simulink model "Quad_Nonlinear_Yaw_PID"  (R2020a)
settings: Solver=ode4  StartTime=0.0  StopTime=10  FixedStep=0.01  RelTol=1e-3
InitFcn:
  | QuadConstants;
undefined symbols (not defined in the file or in its folder): C1, C2, C3, KD_Yaw, KI_Yaw, KP_Yaw, magnitude
libraries: simulink x1
settings Model: Creator=Ali  LastModifiedBy=Ali

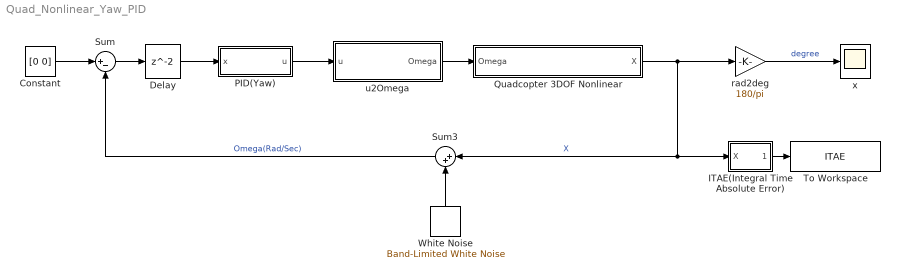
== system Quad_Nonlinear_Yaw_PID ==
  " White Noise" : simulink/Sources/Band-Limited White Noise  Cov=[0.000005]  Ts=.01  seed=[23341]
  Constant : Constant  Value=[0 0]
  Delay : Delay
  ITAE(Integral Time Absolute Error) : Subsystem
  PID(Yaw) : Subsystem
  Quadcopter 3DOF Nonlinear : Subsystem  TreatAsAtomicUnit=on
  Sum : Sum  Inputs=|+-
  Sum3 : Sum  Inputs=|++
  To Workspace : ToWorkspace  VariableName=ITAE  SaveFormat=Timeseries  SampleTime=-1
  rad2deg : Gain  Gain=180/pi
  u2Omega : Subsystem
  x : Scope
  wires:
  Quadcopter 3DOF Nonlinear/1(X) -> Sum3/1, ITAE(Integral Time Absolute Error)/1(X), rad2deg/1  "X"
  ITAE(Integral Time Absolute Error)/1(ITAE) -> To Workspace/1
  " White Noise"/1 -> Sum3/2
  rad2deg/1 -> x/1  "degree"
  Sum3/1 -> Sum/2  "Omega(Rad/Sec)"
  u2Omega/1(Omega) -> Quadcopter 3DOF Nonlinear/1(Omega)
  Constant/1 -> Sum/1
  PID(Yaw)/1(u) -> u2Omega/1(u)
  Sum/1 -> Delay/1
  Delay/1 -> PID(Yaw)/1(x)

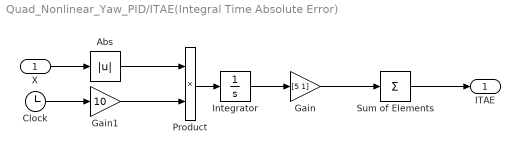
== system Quad_Nonlinear_Yaw_PID/ITAE(Integral Time Absolute Error) ==
  X : Inport
  Abs : Abs
  Clock : Clock
  Gain : Gain  Gain=[5 1]
  Gain1 : Gain  Gain=10
  Integrator : Integrator
  Product : Product
  Sum of Elements : Sum  Inputs=+
  ITAE : Outport
  wires:
  Product/1 -> Integrator/1
  Integrator/1 -> Gain/1
  Clock/1 -> Gain1/1
  Sum of Elements/1 -> ITAE/1
  Abs/1 -> Product/1
  X/1 -> Abs/1
  Gain/1 -> Sum of Elements/1
  Gain1/1 -> Product/2

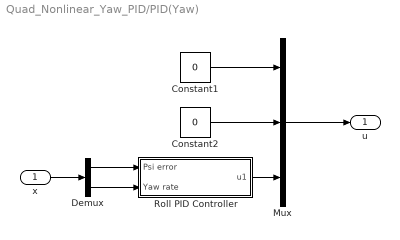
== system Quad_Nonlinear_Yaw_PID/PID(Yaw) ==
  x : Inport
  Constant1 : Constant  Value=0
  Constant2 : Constant  Value=0
  Demux : Demux  Outputs=2
  Mux : Mux  Inputs=3
  Roll PID Controller : Subsystem  VariantControl=Choice
  u : Outport
  wires:
  Mux/1 -> u/1
  x/1 -> Demux/1
  Demux/2 -> Roll PID Controller/2(Yaw rate)
  Demux/1 -> Roll PID Controller/1(Psi error)
  Constant1/1 -> Mux/1
  Roll PID Controller/1(u1) -> Mux/3
  Constant2/1 -> Mux/2

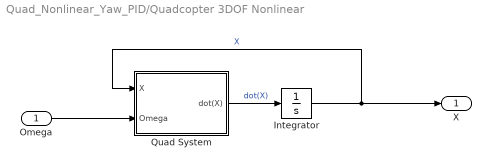
== system Quad_Nonlinear_Yaw_PID/Quadcopter 3DOF Nonlinear ==
  Omega : Inport
  Integrator : Integrator  InitialCondition=[-100*pi/180 -1.2*pi/180]
  Quad System : Subsystem
  X : Outport
  wires:
  Integrator/1 -> Quad System/1(X), X/1  "X"
  Quad System/1(dot(X)) -> Integrator/1  "dot(X)"
  Omega/1 -> Quad System/2(Omega)

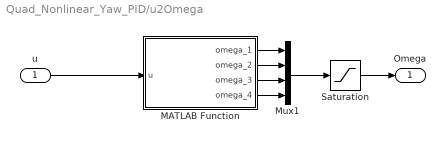
== system Quad_Nonlinear_Yaw_PID/u2Omega ==
  u : Inport
  MATLAB Function : MATLAB Function  TreatAsAtomicUnit=on
  Mux1 : Mux
  Saturation : Saturate  UpperLimit=4000/60*2*pi  LowerLimit=1500/60*2*pi
  Omega : Outport
  wires:
  MATLAB Function/2(omega_2) -> Mux1/2
  u/1 -> MATLAB Function/1(u)
  MATLAB Function/3(omega_3) -> Mux1/3
  MATLAB Function/1(omega_1) -> Mux1/1
  MATLAB Function/4(omega_4) -> Mux1/4
  Mux1/1 -> Saturation/1
  Saturation/1 -> Omega/1

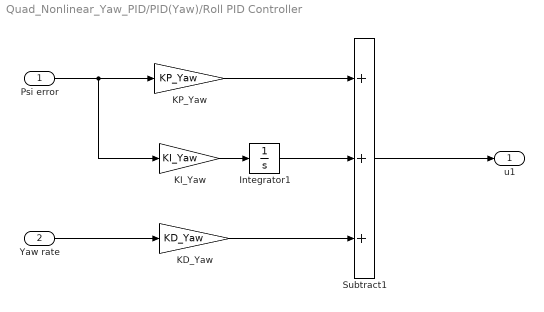
== system Quad_Nonlinear_Yaw_PID/PID(Yaw)/Roll PID Controller ==
  Psi error : Inport
  Yaw rate : Inport  Port=2
  Integrator1 : Integrator
  KD_Yaw : Gain  Gain=KD_Yaw
  KI_Yaw : Gain  Gain=KI_Yaw
  KP_Yaw : Gain  Gain=KP_Yaw
  Subtract1 : Sum  Inputs=+++
  u1 : Outport
  wires:
  Integrator1/1 -> Subtract1/2
  KI_Yaw/1 -> Integrator1/1
  KD_Yaw/1 -> Subtract1/3
  Subtract1/1 -> u1/1
  KP_Yaw/1 -> Subtract1/1
  Yaw rate/1 -> KD_Yaw/1
  Psi error/1 -> KI_Yaw/1, KP_Yaw/1

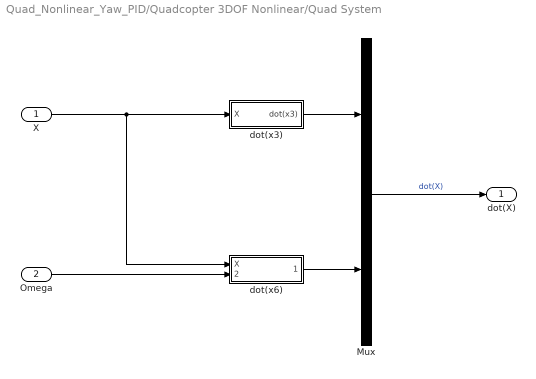
== system Quad_Nonlinear_Yaw_PID/Quadcopter 3DOF Nonlinear/Quad System ==
  X : Inport
  Omega : Inport  Port=2
  Mux : Mux  Inputs=2
  dot(x3) : Subsystem
  dot(x6) : Subsystem
  dot(X) : Outport
  wires:
  Mux/1 -> dot(X)/1  "dot(X)"
  Omega/1 -> dot(x6)/2(Omega)
  dot(x3)/1(dot(x3)) -> Mux/1
  dot(x6)/1(dot(x6)) -> Mux/2
  X/1 -> dot(x6)/1(X), dot(x3)/1(X)

== system Quad_Nonlinear_Yaw_PID/Quadcopter 3DOF Nonlinear/Quad System/dot(x3) ==
  X : Inport
  Subsystem : Subsystem
  dot(x3) : Outport
  wires:
  X/1 -> Subsystem/1(X)
  Subsystem/1(x6cos(x1)) -> dot(x3)/1

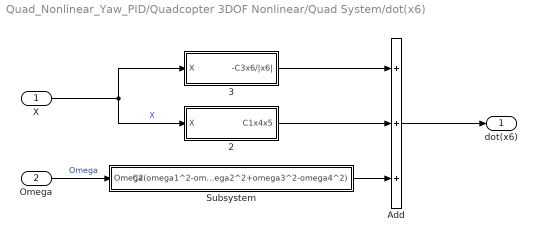
== system Quad_Nonlinear_Yaw_PID/Quadcopter 3DOF Nonlinear/Quad System/dot(x6) ==
  X : Inport
  Omega : Inport  Port=2
  2 : Subsystem
  3 : Subsystem
  Add : Sum  Inputs=+++
  Subsystem : Subsystem
  dot(x6) : Outport
  wires:
  Omega/1 -> Subsystem/1(Omega)  "Omega"
  Add/1 -> dot(x6)/1
  3/1("-C3x6/|x6| ") -> Add/1
  2/1(C1x4x5) -> Add/2
  Subsystem/1(C2(omega1^2-omega2^2+omega3^2-omega4^2)) -> Add/3
  X/1 -> 3/1(X), 2/1(X)  "X"

== system Quad_Nonlinear_Yaw_PID/Quadcopter 3DOF Nonlinear/Quad System/dot(x3)/Subsystem ==
  X : Inport
  Selector : Selector  InputPortWidth=2  IndexOptions=Index vector (dialog)  Indices=[2]  OutputSizes=1
  Subsystem1 : Subsystem
  x6cos(x1) : Outport
  wires:
  Subsystem1/1(x6cos(x1)) -> x6cos(x1)/1  "x6cos(x1)"
  X/1 -> Selector/1  "X"
  Selector/1 -> Subsystem1/1(x6)

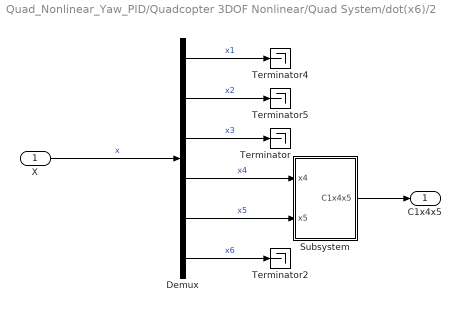
== system Quad_Nonlinear_Yaw_PID/Quadcopter 3DOF Nonlinear/Quad System/dot(x6)/2 ==
  X : Inport
  Demux : Demux  Outputs=6
  Subsystem : Subsystem
  Terminator{,2,4..5} (4 alike) : Terminator
  C1x4x5 : Outport
  wires:
  Demux/4 -> Subsystem/1(x4)  "x4"
  X/1 -> Demux/1  "x"
  Demux/3 -> Terminator/1  "x3"
  Subsystem/1(C1x4x5) -> C1x4x5/1
  Demux/1 -> Terminator4/1  "x1"
  Demux/2 -> Terminator5/1  "x2"
  Demux/5 -> Subsystem/2(x5)  "x5"
  Demux/6 -> Terminator2/1  "x6"

== system Quad_Nonlinear_Yaw_PID/Quadcopter 3DOF Nonlinear/Quad System/dot(x6)/3 ==
  X : Inport
  Selector : Selector  InputPortWidth=2  IndexOptions=Index vector (dialog)  Indices=[2]  OutputSizes=1
  Subsystem : Subsystem
  "-C3x6/|x6| " : Outport
  wires:
  X/1 -> Selector/1  "x"
  Selector/1 -> Subsystem/1(x6)  "x6"
  Subsystem/1("-C3x6/|x6| ") -> "-C3x6/|x6| "/1

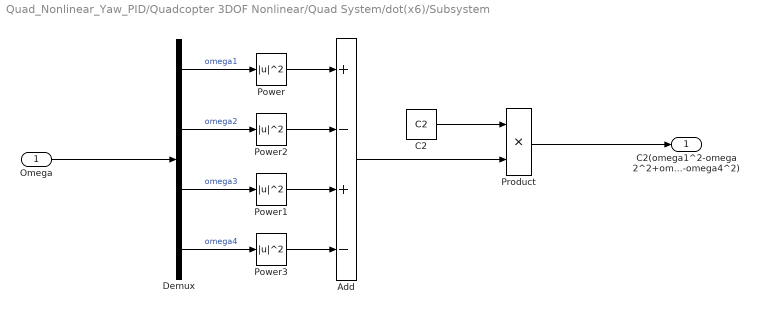
== system Quad_Nonlinear_Yaw_PID/Quadcopter 3DOF Nonlinear/Quad System/dot(x6)/Subsystem ==
  Omega : Inport
  Add : Sum  Inputs=+-+-
  C2 : Constant  Value=C2
  Demux : Demux
  Power{,1..3} (4 alike) : Math  Operator=magnitude^2  SaturateOnIntegerOverflow=on
  Product : Product
  C2(omega1^2-omega2^2+omega3^2-omega4^2) : Outport
  wires:
  Omega/1 -> Demux/1
  Demux/3 -> Power1/1  "omega3"
  Demux/1 -> Power/1  "omega1"
  Demux/2 -> Power2/1  "omega2"
  Demux/4 -> Power3/1  "omega4"
  C2/1 -> Product/1
  Add/1 -> Product/2
  Product/1 -> C2(omega1^2-omega2^2+omega3^2-omega4^2)/1
  Power/1 -> Add/1
  Power2/1 -> Add/2
  Power1/1 -> Add/3
  Power3/1 -> Add/4

== system Quad_Nonlinear_Yaw_PID/Quadcopter 3DOF Nonlinear/Quad System/dot(x3)/Subsystem/Subsystem1 ==
  x6 : Inport
  x6cos(x1) : Outport
  wires:
  x6/1 -> x6cos(x1)/1

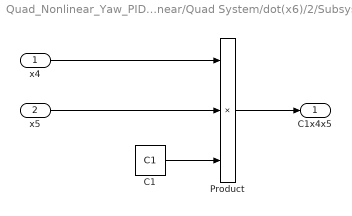
== system Quad_Nonlinear_Yaw_PID/Quadcopter 3DOF Nonlinear/Quad System/dot(x6)/2/Subsystem ==
  x4 : Inport
  x5 : Inport  Port=2
  C1 : Constant  Value=C1
  Product : Product  Inputs=3
  C1x4x5 : Outport
  wires:
  x4/1 -> Product/1
  Product/1 -> C1x4x5/1
  x5/1 -> Product/2
  C1/1 -> Product/3

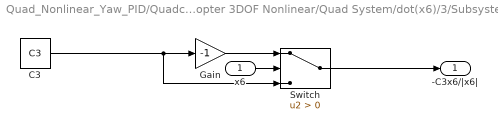
== system Quad_Nonlinear_Yaw_PID/Quadcopter 3DOF Nonlinear/Quad System/dot(x6)/3/Subsystem ==
  x6 : Inport
  C3 : Constant  Value=C3
  Gain : Gain  Gain=-1
  Switch : Switch  Criteria=u2 > Threshold
  "-C3x6/|x6| " : Outport
  wires:
  Switch/1 -> "-C3x6/|x6| "/1
  C3/1 -> Switch/3, Gain/1
  x6/1 -> Switch/2
  Gain/1 -> Switch/1

== matlab function Quad_Nonlinear_Yaw_PID/u2Omega/MATLAB Function ==
  data: u input size=3; omega_1 output size=1; omega_2 output size=1; omega_3 output size=1; omega_4 output size=1
function [omega_1, omega_2, omega_3, omega_4] = fcn(u)
u1 = u(1);
u2 = u(2);
u3 = u(3);
% control effort
u4 = ones(1, length(u1)) * 4 * rpm2rad_sec(2000)^2;
% calculate omega
if (u4 + u3 + 2 * u2) / 4 > 0
    omega_1 = sqrt((u4 + u3 + 2 * u2) / 4);
else
    omega_1 = 0;
end
if (u4 + u3 - 2 * u2) / 4 > 0
    omega_3 = sqrt((u4 + u3 - 2 * u2) / 4);
else
    omega_3 = 0;
end
if (u4 - u3 + 2 * u1) / 4 > 0
    omega_2 = sqrt((u4 - u3 + 2 * u1) / 4);
else
    omega_2 = 0;
end
if (u4 - u3 - 2 * u1) / 4 > 0
    omega_4 = sqrt((u4 - u3 - 2 * u1) / 4);
else
    omega_4 = 0;
end
end
%% functions
% rpm to rad/sec
function rad = rpm2rad_sec(rpm)
rad = rpm / 60 * 2 * pi;
end
